simulink model "Decision_Module_withHistory"  (R2015a)
settings: Solver=FixedStepDiscrete  StartTime=0.0  StopTime=10.0  FixedStep=delta_t  RelTol=1e-3
undefined symbols (not defined in the file): D, delta_t, I, Kd, Kp, M_tilde, psi_dot_max, psi_max, S, S_pinv
settings Model: Creator=Kerianne  LastModifiedBy=Kerianne
settings DataIOCC: SaveFormat=Structure
settings OptimizationCC: InlineParams=on  ExpressionDepthLimit=2147483647
settings DebuggingCC: UnderspecifiedInitializationDetection=Classic  MergeDetectMultiDrivingBlocksExec=none  SolverPrmCheckMsg=warning  StateNameClashWarn=warning

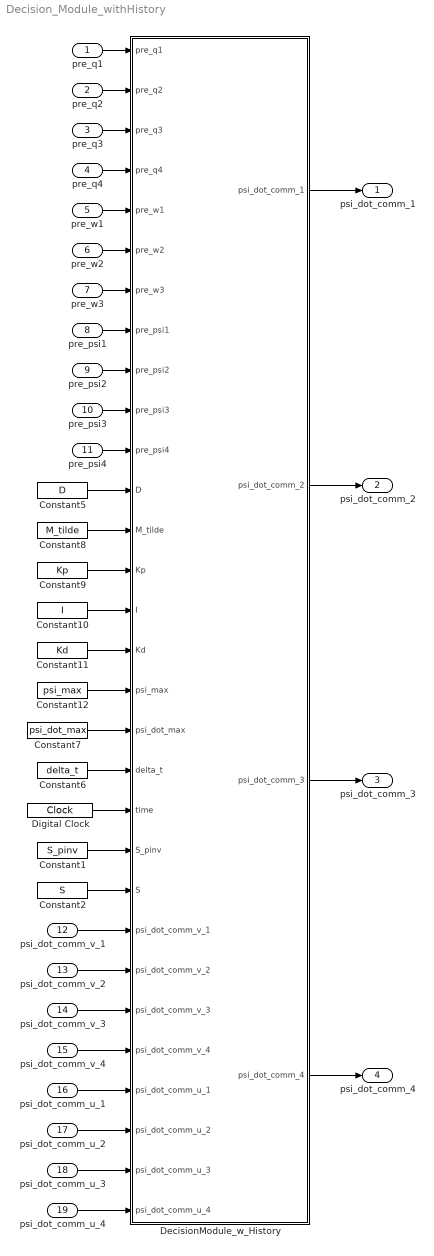
== system Decision_Module_withHistory ==
  pre_q1 : Inport
  pre_q2 : Inport  Port=2
  pre_q3 : Inport  Port=3
  pre_q4 : Inport  Port=4
  pre_w1 : Inport  Port=5
  pre_w2 : Inport  Port=6
  pre_w3 : Inport  Port=7
  pre_psi1 : Inport  Port=8
  pre_psi2 : Inport  Port=9
  pre_psi3 : Inport  Port=10
  pre_psi4 : Inport  Port=11
  psi_dot_comm_v_1 : Inport  Port=12
  psi_dot_comm_v_2 : Inport  Port=13
  psi_dot_comm_v_3 : Inport  Port=14
  psi_dot_comm_v_4 : Inport  Port=15
  psi_dot_comm_u_1 : Inport  Port=16
  psi_dot_comm_u_2 : Inport  Port=17
  psi_dot_comm_u_3 : Inport  Port=18
  psi_dot_comm_u_4 : Inport  Port=19
  Constant1 : Constant  Value=S_pinv
  Constant10 : Constant  Value=I
  Constant11 : Constant  Value=Kd
  Constant12 : Constant  Value=psi_max
  Constant2 : Constant  Value=S
  Constant5 : Constant  Value=D
  Constant6 : Constant  Value=delta_t
  Constant7 : Constant  Value=psi_dot_max
  Constant8 : Constant  Value=M_tilde
  Constant9 : Constant  Value=Kp
  DecisionModule_w_History : MATLAB Function  TreatAsAtomicUnit=on
  Digital Clock : DigitalClock  SampleTime=delta_t
  psi_dot_comm_1 : Outport
  psi_dot_comm_2 : Outport  Port=2
  psi_dot_comm_3 : Outport  Port=3
  psi_dot_comm_4 : Outport  Port=4
  wires:
  Constant6/1 -> DecisionModule_w_History/19(delta_t)
  Constant7/1 -> DecisionModule_w_History/18(psi_dot_max)
  Constant12/1 -> DecisionModule_w_History/17(psi_max)
  Constant11/1 -> DecisionModule_w_History/16(Kd)
  Constant10/1 -> DecisionModule_w_History/15(I)
  Constant9/1 -> DecisionModule_w_History/14(Kp)
  Constant8/1 -> DecisionModule_w_History/13(M_tilde)
  Constant5/1 -> DecisionModule_w_History/12(D)
  pre_psi3/1 -> DecisionModule_w_History/10(pre_psi3)
  pre_psi2/1 -> DecisionModule_w_History/9(pre_psi2)
  pre_psi1/1 -> DecisionModule_w_History/8(pre_psi1)
  pre_w3/1 -> DecisionModule_w_History/7(pre_w3)
  pre_w2/1 -> DecisionModule_w_History/6(pre_w2)
  pre_w1/1 -> DecisionModule_w_History/5(pre_w1)
  pre_q4/1 -> DecisionModule_w_History/4(pre_q4)
  pre_q3/1 -> DecisionModule_w_History/3(pre_q3)
  pre_q2/1 -> DecisionModule_w_History/2(pre_q2)
  pre_q1/1 -> DecisionModule_w_History/1(pre_q1)
  DecisionModule_w_History/3(psi_dot_comm_3) -> psi_dot_comm_3/1
  DecisionModule_w_History/1(psi_dot_comm_1) -> psi_dot_comm_1/1
  DecisionModule_w_History/2(psi_dot_comm_2) -> psi_dot_comm_2/1
  Constant1/1 -> DecisionModule_w_History/21(S_pinv)
  DecisionModule_w_History/4(psi_dot_comm_4) -> psi_dot_comm_4/1
  pre_psi4/1 -> DecisionModule_w_History/11(pre_psi4)
  Constant2/1 -> DecisionModule_w_History/22(S)
  psi_dot_comm_v_1/1 -> DecisionModule_w_History/23(psi_dot_comm_v_1)
  psi_dot_comm_v_2/1 -> DecisionModule_w_History/24(psi_dot_comm_v_2)
  psi_dot_comm_v_3/1 -> DecisionModule_w_History/25(psi_dot_comm_v_3)
  psi_dot_comm_v_4/1 -> DecisionModule_w_History/26(psi_dot_comm_v_4)
  psi_dot_comm_u_1/1 -> DecisionModule_w_History/27(psi_dot_comm_u_1)
  psi_dot_comm_u_2/1 -> DecisionModule_w_History/28(psi_dot_comm_u_2)
  psi_dot_comm_u_3/1 -> DecisionModule_w_History/29(psi_dot_comm_u_3)
  psi_dot_comm_u_4/1 -> DecisionModule_w_History/30(psi_dot_comm_u_4)
  Digital Clock/1 -> DecisionModule_w_History/20(time)

== matlab function Decision_Module_withHistory/DecisionModule_w_History ==
  data: pre_q1 input; pre_q2 input; pre_q3 input; pre_q4 input; pre_w1 input; pre_w2 input; pre_w3 input; pre_psi1 input; pre_psi2 input; pre_psi3 input; pre_psi4 input; psi_dot_comm_1 output; D input; M_tilde input; Kp input; I input; Kd input; psi_max input; psi_dot_max input; delta_t input; time input; psi_dot_comm_2 output; psi_dot_comm_3 output; psi_dot_comm_4 output; S_pinv input; S input; psi_dot_comm_v_1 input; psi_dot_comm_v_2 input; psi_dot_comm_v_3 input; psi_dot_comm_v_4 input; psi_dot_comm_u_1 input; psi_dot_comm_u_2 input; psi_dot_comm_u_3 input; psi_dot_comm_u_4 input
function [psi_dot_comm_1, psi_dot_comm_2, psi_dot_comm_3,psi_dot_comm_4] = fcn(pre_q1,pre_q2,pre_q3,pre_q4,pre_w1,pre_w2,pre_w3,pre_psi1,pre_psi2,pre_psi3,pre_psi4,D,M_tilde,Kp,I,Kd,psi_max,psi_dot_max,delta_t,time,S_pinv,S,psi_dot_comm_v_1,psi_dot_comm_v_2,psi_dot_comm_v_3,psi_dot_comm_v_4,psi_dot_comm_u_1,psi_dot_comm_u_2,psi_dot_comm_u_3,psi_dot_comm_u_4)
% Decision Module for Reaction Wheel Control
% Author: Kerianne Gross, AFRL/RQQA, kerianne.gross@us.af.mil
% Last Updated: 
% 20 November 2015 
%
% This version of the decision module checks to see whether the unverified
% controller has violated the safety properties in a previous time step.
% Thought being that if the saftey properties have been violated
% previously, then the unverified controller cannot be trusted.
%
% This is a decision module that takes in the current state of the
% spacecraft, the outputs of the verified PID controller, and the outputs
% of the unverified blackbox controller and determines which controller
% signals make it out.
% 1) Check to see if unverified commanded acceleration (psi_dot_comm_u_x)
%    is > than max commanded acceleration (psi_dot_max) for any of the 
%    wheels. IF acceleration boundary is VIOLATED (psi_dot_comm_u_x > 
%    psi_dot_max),then use verified commanded acceleration signal  
%    (psi_dot_comm_v_x) for all wheels. 
% 2) Check to see if unverified commanded acceleration (psi_dot_comm_u_x)
%    would cause the wheel velocity (psi(x) to exceend the max velocity 
%    (psi_max) for any of the wheels. IF acceleration boundary is VIOLATED,
%    then use verified commanded acceleration signal (psi_dot_comm_v_x) for 
%    all wheels.
% 3) If none of the above conditions are violated, use the unverified
%    signal
% 
% DISCUSSION
%  > Why not just switch out the 1 bad signal, rather than all of the 
%    signals? Well, if one signal is 
%    bad, the unverified controller is no longer considered trustworthy 
%    until all signals are in bounds again. Depending on the criticality of 
%    the signal, one may want to add a flag to show that a violation 
%    occurred and use a different switching mechanism to switch back.
%  > There may be other characteristics you are trying to protect against
%    too, for instance, maybe you don't wan the spacecraft angular velocity
%    (w) to exceed a threshold, because it would make it very difficult to
%    recover beyond that threshold. These conditions just need to be listed
%    in order of precedence.
     % States at the end fot he last time step
    q       = [pre_q1,pre_q2,pre_q3,pre_q4];    %s/c quaternion
    omega   = [pre_w1,pre_w2,pre_w3];           %s/c angular rates 
    psi     = [pre_psi1,pre_psi2,pre_psi3,pre_psi4];     %RWA angle rates
        
    % Use persistent variable Violation to keep time history of the system
    persistent Violation
    if isempty(Violation)
        Violation = 0;
    end
    
    % CHECKS: 1) PREVIOUS VIOLATION
    %         2) VIOLATION OF RW MAX ANGULAR ACCELERATION (PSI_DOT_MAX)
    %         2) VIOLATION OF RW MAX ANGULAR VELOCITY (PSI_MAX)
    if (Violation == 1 || ...
        abs(psi_dot_comm_u_1) > psi_dot_max || ...
        abs(psi_dot_comm_u_2) > psi_dot_max || ...
        abs(psi_dot_comm_u_3) > psi_dot_max || ...
        abs(psi_dot_comm_u_4) > psi_dot_max || ...
        abs(psi(1)+ psi_dot_comm_u_1*delta_t) > psi_max || ...
        abs(psi(2)+ psi_dot_comm_u_2*delta_t) > psi_max || ...
        abs(psi(3)+ psi_dot_comm_u_3*delta_t) > psi_max || ...
        abs(psi(4)+ psi_dot_comm_u_4*delta_t) > psi_max)
        Violation_flag = 1;
    else
        Violation_flag = 0;
    end
    % CHECK: PREVIOUSLY VIOLATED
    if (Violation_flag == 1)
        psi_dot_comm_1 = psi_dot_comm_v_1;
        psi_dot_comm_2 = psi_dot_comm_v_2;
        psi_dot_comm_3 = psi_dot_comm_v_3;
        psi_dot_comm_4 = psi_dot_comm_v_4; 
    else
        psi_dot_comm_1 = psi_dot_comm_u_1;
        psi_dot_comm_2 = psi_dot_comm_u_2;
        psi_dot_comm_3 = psi_dot_comm_u_3;
        psi_dot_comm_4 = psi_dot_comm_u_4;
    end

% Keep record if Violation has occured
if Violation_flag == 1
    Violation = Violation_flag;
end
